simulink library "vmc"  (R2021b)
settings: Solver=VariableStepAuto  StartTime=0.0  StopTime=10.0  RelTol=1e-3
undefined symbols (not defined in the file or in its folder): AVMC_ACCDeltaTqIGain_X_kph, AVMC_ACCDeltaTqIGain_Y_mps2, AVMC_ACCDeltaTqIGainP2_X_kph, AVMC_ACCDeltaTqIGainP2_Y_mps2, AVMC_ACCDeltaTqPGain_X_kph, AVMC_ACCDeltaTqPGain_Y_kph, AVMC_ACCDeltaTqPGainP2_X_kph, AVMC_ACCDeltaTqPGainP2_Y_kph, AVMC_ACCLongSteadyCtrl_X_kph, AVMC_CCAccelCMD_X_kph, AVMC_CCAccelCMD_Y_kph, AVMC_CCDeltaTqIGain_X_kph, AVMC_CCDeltaTqIGain_Y_mps2, AVMC_CCDeltaTqPGain_X_kph, AVMC_CCDeltaTqPGain_Y_kph, AVMC_CCLongSteadyCtrl_X_kph, AVMC_DISCDeltaTqIGainP2_X_kph, AVMC_DISCDeltaTqIGainP2_Y_mps2, AVMC_ESCRegenOut_X_kph, AVMC_ESCRegenOut_Y_Deg, AVMC_ESCRegenOutEnSpd_X_Deg, AVMC_LatESCRegenOut_X_kph, AVMC_LatESCRegenOut_Y_Deg, AVMC_LongAccDeadZone_X_kph, AVMC_LongAccDeadZoneP2_X_kph, AVMC_LongAccFiltTs_X_Gps, AVMC_LongAccFiltTsP2_X_Gps, AVMC_MCPresBaseTq_X_bar, AVMC_MSAAccelCMD_X_kph, AVMC_MSAAccelCMD_Y_kph, AVMC_MSADeltaTqIGain_X_kph, AVMC_MSADeltaTqIGain_Y_mps2, AVMC_MSADeltaTqPGain_X_kph, AVMC_MSADeltaTqPGain_Y_kph, AVMC_MSALongSteadyCtrl_X_kph, AVMC_MSAPedalOvrd_X_kph, AVMC_MSASpdBand_X_kph, AVMC_OPDDisSlideRate_X_Deg, AVMC_RDCDetectTime_X_kph, AVMC_RDCDetectTime_Y_pct, AVMC_RDCEnSlideRate_X_Deg, AVMC_StESCYaw_X_kph, AVMC_StESCYaw_Y_Deg, AVMC_StESCYawCom_X_kph, AVMC_StESCYawCom_Y_Gps, AVMC_TMSpdBaseTq_X_rpm, C_TASK_10MS_S, C_TASK_5MS_S, DEG2RAD, Discrete, ENUM_ADASACCSTA_ACTIVE, ENUM_ADASACCSTA_OVERRIDE, ENUM_ADASACCSTA_STANDBY, ENUM_ADASMSASTA_ACTIVE, ENUM_ADASMSASTA_ERROR, ENUM_ADASMSASTA_OFF, ENUM_ADASMSASTA_OVERSPEED, ENUM_ADASMSASTA_STANDBY, ENUM_ADASMSASTA_UNDERSPEED, ENUM_ADASMSASTA_UNLIMIT ... (+254)
libraries: hcu_lib x57, simulink x49, ctrlSharedLib x6, simulink_extras x1
(part 8 of 9)

== system vmc/VMC/Slide Rate  Calculation/4Wheel Calculation/LR Wheel ==
  VVMC_4WheelLongAcc_Gps : Inport
  task_time_s : Inport  Port=2
  VINP_LRRawWhlSpeed_kph : Inport  Port=3
  VTQD_GearActualPosn_enum : Inport  Port=4
  AND3 : Logic  Inputs=3  AllPortsSameDT=off  OutDataTypeStr=boolean
  Abs2 : Abs
  Add : Sum
  Add{4,7,13..14} (4 alike) : Sum  Inputs=+-
  Constant1 : Constant  Value=GRAVITY_G
  Constant11 : Constant  Value=KPH2MPS
  Constant19 : Constant  Value=ONE_PERCENT
  Constant2 : Constant  Value=MPS2KPH
  Constant20 : Constant  Value=KVMC_RawWhlSpeedDeadZone_kph
  Constant21 : Constant  Value=ZERO_FLOAT
  Constant22 : Constant  Value=KVMC_RawWhlSpeedDeadZone_kph
  Constant23 : Constant  Value=ONE_FLOAT
  Constant30 : Constant  Value=KPH2MPS
  Constant31 : Constant  Value=GRAVITY_G
  Constant32 : Constant  Value=KVMC_WhlSpdCalAccTs_c
  Constant40 : Constant  Value=KVMC_WheelSkidAccDev_Gps
  Constant41 : Constant  Value=KVMC_SkidRecVehSpdDev_kph
  Constant44 : Constant  Value=KPH2MPS
  Constant46 : Constant  Value=ENUM_GEARACTUALPOSN_D
  Constant47 : Constant  Value=ENUM_GEARACTUALPOSN_R
  Constant48 : Constant  Value=KVMC_PreVehSpdCalSW_flg
  Constant5 : Constant  Value=KVMC_4WheelEnSkidDetSpd_kph
  Constant50 : Constant  Value=KVMC_LRWhlSkidReset_flg
  Delay{,3,5,10..11,16} (6 alike) : Delay  DelayLength=1
  Divide4 : Product  Inputs=*//
  Divide6 : Product  Inputs=**//
  Equal : RelationalOperator  Operator===  OutDataTypeStr=boolean  RndMeth=Simplest
  Equal1 : RelationalOperator  Operator===  OutDataTypeStr=boolean  RndMeth=Simplest
  FirstOrderFilter2 : hcu_lib/Basic_Blocks/FirstOrderFilter
  OR : Logic  Operator=OR  AllPortsSameDT=off  OutDataTypeStr=boolean
  OR1 : Logic  Operator=OR  AllPortsSameDT=off  OutDataTypeStr=boolean
  OR2 : Logic  Operator=OR  AllPortsSameDT=off  OutDataTypeStr=boolean
  Product : Product
  Product1 : Product  Inputs=3
  Product2 : Product
  Product3 : Product
  Relational Operator12 : RelationalOperator  Operator=>  OutDataTypeStr=boolean  RndMeth=Simplest
  Relational Operator{2,7..8,13} (4 alike) : RelationalOperator  Operator=<=  OutDataTypeStr=boolean  RndMeth=Simplest
  SR_Latch2 : hcu_lib/Basic_Blocks/SR_Latch
  Saturation : Saturate  UpperLimit=KVMC_PredVehSpdLimit_mps  LowerLimit=ZERO_FLOAT
  Switch{,7..8,10} (4 alike) : Switch  Criteria=u2 > Threshold
  VVMC_LRPreVehSpd_kph : Outport
  VVMC_LRWhlSkid_flg : Outport  Port=2
  VVMC_LR4WhlSpdSlideRate_pct : Outport  Port=3
  wires:
  Delay3/1 -> Add7/2
  Delay10/1 -> Add13/1
  Constant30/1 -> Divide6/2
  [task_time_s] -> Divide6/3
  Constant41/1 -> Relational Operator13/2
  Constant50/1 -> AND3/3
  Constant31/1 -> Divide6/4
  [VINP_LRRawWhlSpeed_kph] -> Delay11/1
  SR_Latch2/1 -> [VVMC_LRWhlSkid_flg]  "VVMC_LRWhlSkid_flg"
  [VVMC_LRWhlSkid_flg] -> Delay16/1
  Relational Operator13/1 -> AND3/1
  Abs2/1 -> Relational Operator13/1
  Delay16/1 -> AND3/2
  Add7/1 -> Divide6/1
  Relational Operator12/1 -> SR_Latch2/1
  Delay11/1 -> Add13/2
  [VINP_LRRawWhlSpeed_kph] -> Add7/1
  [VINP_LRRawWhlSpeed_kph] -> Delay3/1
  [VVMC_LRWhlCalAcc_Gps] -> Add14/1
  Constant32/1 -> FirstOrderFilter2/3
  FirstOrderFilter2/1 -> [VVMC_LRWhlCalAcc_Gps]  "VVMC_LRWhlCalAcc_Gps"
  Divide6/1 -> FirstOrderFilter2/1
  [VVMC_4WheelLongAcc_Gps] -> Add14/2
  Constant40/1 -> Relational Operator12/2
  Add13/1 -> Abs2/1
  Add14/1 -> Relational Operator12/1
  [task_time_s] -> FirstOrderFilter2/2
  [VVMC_LRPreVehSpd_kph] -> Delay5/1
  [task_time_s] -> Product1/3
  [VVMC_4WheelLongAcc_Gps] -> Product1/1
  Constant44/1 -> Product3/2
  Switch/1 -> Saturation/1  "VVMC_LRLastPreVehSpd_mps"
  Product2/1 -> Switch10/1
  Constant11/1 -> Product/2
  Add/1 -> Product2/1  "VVMC_LRCalPreVehSpd_mps"
  Equal/1 -> OR/1
  [VTQD_GearActualPosn_enum] -> Equal/1
  [VINP_LRRawWhlSpeed_kph] -> Switch10/3
  Constant1/1 -> Product1/2
  Product3/1 -> Switch/1
  Switch10/1 -> [VVMC_LRPreVehSpd_kph]  "VVMC_LRPreVehSpd_kph"
  [VINP_LRRawWhlSpeed_kph] -> Delay/1
  OR1/1 -> Switch/2
  Constant48/1 -> OR1/2
  Constant47/1 -> Equal1/2
  Equal1/1 -> OR/2
  [VTQD_GearActualPosn_enum] -> Equal1/1
  Constant46/1 -> Equal/2
  Constant2/1 -> Product2/2
  Product1/1 -> Add/1  "VVMC_LRDeltaVehSpd_mps"
  Delay/1 -> Product/1
  Product/1 -> Switch/3
  Delay5/1 -> Product3/1
  Saturation/1 -> Add/2
  OR/1 -> Switch10/2
  [VVMC_LRWhlSkid_flg] -> OR1/1
  [VVMC_LRPreVehSpd_kph] -> Delay10/1
  Constant22/1 -> Relational Operator7/2
  [VINP_LRRawWhlSpeed_kph] -> Add4/1
  [VINP_LRRawWhlSpeed_kph] -> Relational Operator8/1
  Relational Operator7/1 -> Switch7/2
  [VVMC_LRPreVehSpd_kph] -> Relational Operator7/1
  Constant19/1 -> Divide4/2
  Switch8/1 -> [VVMC_LR4WhlSpdSlideRate_pct]  "VVMC_LR4WhlSpdSlideRate_pct"
  Constant23/1 -> Switch7/1
  [VVMC_LRPreVehSpd_kph] -> Add4/2
  Constant20/1 -> Relational Operator8/2
  Constant21/1 -> Switch8/1
  Divide4/1 -> Switch8/3  "VVMC_LRCal4WhlSpdSlideRate_pct"
  Switch7/1 -> Divide4/3
  [VVMC_LRPreVehSpd_kph] -> Switch7/3
  Add4/1 -> Divide4/1
  Relational Operator8/1 -> Switch8/2
  task_time_s/1 -> [task_time_s]
  VVMC_4WheelLongAcc_Gps/1 -> [VVMC_4WheelLongAcc_Gps]
  VINP_LRRawWhlSpeed_kph/1 -> [VINP_LRRawWhlSpeed_kph]
  VTQD_GearActualPosn_enum/1 -> [VTQD_GearActualPosn_enum]
  [VVMC_LRPreVehSpd_kph] -> VVMC_LRPreVehSpd_kph/1
  [VVMC_LRWhlSkid_flg] -> VVMC_LRWhlSkid_flg/1
  [VVMC_LR4WhlSpdSlideRate_pct] -> VVMC_LR4WhlSpdSlideRate_pct/1
  [VINP_LRRawWhlSpeed_kph] -> Relational Operator2/1
  Relational Operator2/1 -> OR2/1
  Constant5/1 -> Relational Operator2/2
  AND3/1 -> OR2/2
  OR2/1 -> SR_Latch2/2  "VVMC_LRWhlSkidReset_flg"

== system vmc/VMC/Slide Rate  Calculation/4Wheel Calculation/RF Wheel ==
  VVMC_4WheelLongAcc_Gps : Inport
  task_time_s : Inport  Port=2
  VINP_RFRawWhlSpeed_kph : Inport  Port=3
  VTQD_GearActualPosn_enum : Inport  Port=4
  AND2 : Logic  Inputs=3  AllPortsSameDT=off  OutDataTypeStr=boolean
  Abs1 : Abs
  Add : Sum
  Add{2,6,11..12} (4 alike) : Sum  Inputs=+-
  Constant1 : Constant  Value=GRAVITY_G
  Constant10 : Constant  Value=ONE_PERCENT
  Constant11 : Constant  Value=KPH2MPS
  Constant12 : Constant  Value=KVMC_RawWhlSpeedDeadZone_kph
  Constant13 : Constant  Value=ZERO_FLOAT
  Constant2 : Constant  Value=MPS2KPH
  Constant27 : Constant  Value=KPH2MPS
  Constant28 : Constant  Value=GRAVITY_G
  Constant29 : Constant  Value=KVMC_WhlSpdCalAccTs_c
  Constant3 : Constant  Value=KVMC_RawWhlSpeedDeadZone_kph
  Constant38 : Constant  Value=KVMC_WheelSkidAccDev_Gps
  Constant39 : Constant  Value=KVMC_SkidRecVehSpdDev_kph
  Constant4 : Constant  Value=ONE_FLOAT
  Constant44 : Constant  Value=KPH2MPS
  Constant46 : Constant  Value=ENUM_GEARACTUALPOSN_D
  Constant47 : Constant  Value=ENUM_GEARACTUALPOSN_R
  Constant48 : Constant  Value=KVMC_PreVehSpdCalSW_flg
  Constant5 : Constant  Value=KVMC_4WheelEnSkidDetSpd_kph
  Constant51 : Constant  Value=KVMC_RFWhlSkidReset_flg
  Delay{,2,5,8..9,15} (6 alike) : Delay  DelayLength=1
  Divide2 : Product  Inputs=*//
  Divide5 : Product  Inputs=**//
  Equal : RelationalOperator  Operator===  OutDataTypeStr=boolean  RndMeth=Simplest
  Equal1 : RelationalOperator  Operator===  OutDataTypeStr=boolean  RndMeth=Simplest
  FirstOrderFilter1 : hcu_lib/Basic_Blocks/FirstOrderFilter
  OR : Logic  Operator=OR  AllPortsSameDT=off  OutDataTypeStr=boolean
  OR1 : Logic  Operator=OR  AllPortsSameDT=off  OutDataTypeStr=boolean
  OR2 : Logic  Operator=OR  AllPortsSameDT=off  OutDataTypeStr=boolean
  Product : Product
  Product1 : Product  Inputs=3
  Product2 : Product
  Product3 : Product
  Relational Operator{1..2,4,11} (4 alike) : RelationalOperator  Operator=<=  OutDataTypeStr=boolean  RndMeth=Simplest
  Relational Operator10 : RelationalOperator  Operator=>  OutDataTypeStr=boolean  RndMeth=Simplest
  SR_Latch1 : hcu_lib/Basic_Blocks/SR_Latch
  Saturation : Saturate  UpperLimit=KVMC_PredVehSpdLimit_mps  LowerLimit=ZERO_FLOAT
  Switch{,1,4,10} (4 alike) : Switch  Criteria=u2 > Threshold
  VVMC_RFPreVehSpd_kph : Outport
  VVMC_RFWhlSkid_flg : Outport  Port=2
  VVMC_RF4WhlSpdSlideRate_pct : Outport  Port=3
  wires:
  [VVMC_4WheelLongAcc_Gps] -> Add12/2
  Switch1/1 -> Divide2/3
  Relational Operator11/1 -> AND2/1
  Divide5/1 -> FirstOrderFilter1/1
  Constant12/1 -> Relational Operator4/2
  Add12/1 -> Relational Operator10/1
  [VINP_RFRawWhlSpeed_kph] -> Add6/1
  Constant13/1 -> Switch4/1
  [VINP_RFRawWhlSpeed_kph] -> Delay2/1
  Constant3/1 -> Relational Operator1/2
  Delay15/1 -> AND2/2
  [VVMC_RFWhlSkid_flg] -> Delay15/1
  Constant27/1 -> Divide5/2
  Relational Operator1/1 -> Switch1/2
  Constant28/1 -> Divide5/4
  Add11/1 -> Abs1/1
  Constant38/1 -> Relational Operator10/2
  Divide2/1 -> Switch4/3  "VVMC_RFCal4WhlSpdSlideRate_pct"
  Delay8/1 -> Add11/1
  [VINP_RFRawWhlSpeed_kph] -> Delay9/1
  Abs1/1 -> Relational Operator11/1
  [task_time_s] -> FirstOrderFilter1/2
  Delay9/1 -> Add11/2
  Constant39/1 -> Relational Operator11/2
  Constant4/1 -> Switch1/1
  Relational Operator4/1 -> Switch4/2
  Constant51/1 -> AND2/3
  Add6/1 -> Divide5/1
  Constant10/1 -> Divide2/2
  [VINP_RFRawWhlSpeed_kph] -> Add2/1
  [VINP_RFRawWhlSpeed_kph] -> Relational Operator4/1
  Relational Operator10/1 -> SR_Latch1/1
  SR_Latch1/1 -> [VVMC_RFWhlSkid_flg]  "VVMC_RFWhlSkid_flg"
  [VVMC_RFWhlCalAcc_Gps] -> Add12/1
  Constant29/1 -> FirstOrderFilter1/3
  FirstOrderFilter1/1 -> [VVMC_RFWhlCalAcc_Gps]  "VVMC_RFWhlCalAcc_Gps"
  Switch4/1 -> [VVMC_RF4WhlSpdSlideRate_pct]  "VVMC_RF4WhlSpdSlideRate_pct"
  Add2/1 -> Divide2/1
  Delay2/1 -> Add6/2
  [task_time_s] -> Divide5/3
  Product/1 -> Switch/3
  Delay5/1 -> Product3/1
  Product3/1 -> Switch/1
  [VVMC_RFPreVehSpd_kph] -> Delay5/1
  [VINP_RFRawWhlSpeed_kph] -> Delay/1
  OR/1 -> Switch10/2
  [VTQD_GearActualPosn_enum] -> Equal/1
  [VINP_RFRawWhlSpeed_kph] -> Switch10/3
  [VTQD_GearActualPosn_enum] -> Equal1/1
  Delay/1 -> Product/1
  Saturation/1 -> Add/2
  Constant2/1 -> Product2/2
  Product1/1 -> Add/1  "VVMC_RFDeltaVehSpd_mps"
  Equal1/1 -> OR/2
  Constant46/1 -> Equal/2
  OR1/1 -> Switch/2
  Constant47/1 -> Equal1/2
  Constant48/1 -> OR1/2
  Switch10/1 -> [VVMC_RFPreVehSpd_kph]  "VVMC_RFPreVehSpd_kph"
  Constant1/1 -> Product1/2
  Product2/1 -> Switch10/1
  Constant11/1 -> Product/2
  Switch/1 -> Saturation/1  "VVMC_RFLastPreVehSpd_mps"
  Constant44/1 -> Product3/2
  [VVMC_4WheelLongAcc_Gps] -> Product1/1
  [task_time_s] -> Product1/3
  Equal/1 -> OR/1
  Add/1 -> Product2/1  "VVMC_RFCalPreVehSpd_mps"
  [VVMC_RFWhlSkid_flg] -> OR1/1
  [VVMC_RFPreVehSpd_kph] -> Delay8/1
  [VVMC_RFPreVehSpd_kph] -> Add2/2
  [VVMC_RFPreVehSpd_kph] -> Relational Operator1/1
  [VVMC_RFPreVehSpd_kph] -> Switch1/3
  VTQD_GearActualPosn_enum/1 -> [VTQD_GearActualPosn_enum]
  VINP_RFRawWhlSpeed_kph/1 -> [VINP_RFRawWhlSpeed_kph]
  VVMC_4WheelLongAcc_Gps/1 -> [VVMC_4WheelLongAcc_Gps]
  task_time_s/1 -> [task_time_s]
  [VVMC_RFPreVehSpd_kph] -> VVMC_RFPreVehSpd_kph/1
  [VVMC_RFWhlSkid_flg] -> VVMC_RFWhlSkid_flg/1
  [VVMC_RF4WhlSpdSlideRate_pct] -> VVMC_RF4WhlSpdSlideRate_pct/1
  Constant5/1 -> Relational Operator2/2
  Relational Operator2/1 -> OR2/1
  [VINP_RFRawWhlSpeed_kph] -> Relational Operator2/1
  AND2/1 -> OR2/2
  OR2/1 -> SR_Latch1/2  "VVMC_RFWhlSkidReset_flg"

== system vmc/VMC/Slide Rate  Calculation/4Wheel Calculation/RR Wheel ==
  VVMC_4WheelLongAcc_Gps : Inport
  task_time_s : Inport  Port=2
  VINP_RRRawWhlSpeed_kph : Inport  Port=3
  VTQD_GearActualPosn_enum : Inport  Port=4
  AND4 : Logic  Inputs=3  AllPortsSameDT=off  OutDataTypeStr=boolean
  Abs3 : Abs
  Add : Sum
  Add{3,8,15..16} (4 alike) : Sum  Inputs=+-
  Constant1 : Constant  Value=GRAVITY_G
  Constant11 : Constant  Value=KPH2MPS
  Constant14 : Constant  Value=ONE_PERCENT
  Constant15 : Constant  Value=KVMC_RawWhlSpeedDeadZone_kph
  Constant16 : Constant  Value=ZERO_FLOAT
  Constant17 : Constant  Value=KVMC_RawWhlSpeedDeadZone_kph
  Constant18 : Constant  Value=ONE_FLOAT
  Constant2 : Constant  Value=MPS2KPH
  Constant33 : Constant  Value=KPH2MPS
  Constant34 : Constant  Value=GRAVITY_G
  Constant35 : Constant  Value=KVMC_WhlSpdCalAccTs_c
  Constant42 : Constant  Value=KVMC_WheelSkidAccDev_Gps
  Constant43 : Constant  Value=KVMC_SkidRecVehSpdDev_kph
  Constant44 : Constant  Value=KPH2MPS
  Constant46 : Constant  Value=ENUM_GEARACTUALPOSN_D
  Constant47 : Constant  Value=ENUM_GEARACTUALPOSN_R
  Constant48 : Constant  Value=KVMC_PreVehSpdCalSW_flg
  Constant49 : Constant  Value=KVMC_RRWhlSkidReset_flg
  Constant5 : Constant  Value=KVMC_4WheelEnSkidDetSpd_kph
  Delay{,4..5,12..13,17} (6 alike) : Delay  DelayLength=1
  Divide3 : Product  Inputs=*//
  Divide7 : Product  Inputs=**//
  Equal : RelationalOperator  Operator===  OutDataTypeStr=boolean  RndMeth=Simplest
  Equal1 : RelationalOperator  Operator===  OutDataTypeStr=boolean  RndMeth=Simplest
  FirstOrderFilter3 : hcu_lib/Basic_Blocks/FirstOrderFilter
  OR : Logic  Operator=OR  AllPortsSameDT=off  OutDataTypeStr=boolean
  OR1 : Logic  Operator=OR  AllPortsSameDT=off  OutDataTypeStr=boolean
  OR2 : Logic  Operator=OR  AllPortsSameDT=off  OutDataTypeStr=boolean
  Product : Product
  Product1 : Product  Inputs=3
  Product2 : Product
  Product3 : Product
  Relational Operator14 : RelationalOperator  Operator=>  OutDataTypeStr=boolean  RndMeth=Simplest
  Relational Operator{2,5..6,15} (4 alike) : RelationalOperator  Operator=<=  OutDataTypeStr=boolean  RndMeth=Simplest
  SR_Latch3 : hcu_lib/Basic_Blocks/SR_Latch
  Saturation : Saturate  UpperLimit=KVMC_PredVehSpdLimit_mps  LowerLimit=ZERO_FLOAT
  Switch{,5..6,10} (4 alike) : Switch  Criteria=u2 > Threshold
  VVMC_RRPreVehSpd_kph : Outport
  VVMC_RRWhlSkid_flg : Outport  Port=2
  VVMC_RR4WhlSpdSlideRate_pct : Outport  Port=3
  wires:
  [VINP_RRRawWhlSpeed_kph] -> Add8/1
  Constant49/1 -> AND4/3
  Add8/1 -> Divide7/1
  [task_time_s] -> Divide7/3
  Add15/1 -> Abs3/1
  Relational Operator14/1 -> SR_Latch3/1
  [VVMC_4WheelLongAcc_Gps] -> Add16/2
  [task_time_s] -> FirstOrderFilter3/2
  [VINP_RRRawWhlSpeed_kph] -> Delay4/1
  Constant42/1 -> Relational Operator14/2
  FirstOrderFilter3/1 -> [VVMC_RRWhlCalAcc_Gps]  "VVMC_RRWhlCalAcc_Gps"
  Divide7/1 -> FirstOrderFilter3/1
  Relational Operator15/1 -> AND4/1
  Delay4/1 -> Add8/2
  Delay17/1 -> AND4/2
  [VVMC_RRWhlSkid_flg] -> Delay17/1
  Add16/1 -> Relational Operator14/1
  Delay12/1 -> Add15/1
  Constant43/1 -> Relational Operator15/2
  Delay13/1 -> Add15/2
  Constant33/1 -> Divide7/2
  Constant34/1 -> Divide7/4
  Abs3/1 -> Relational Operator15/1
  SR_Latch3/1 -> [VVMC_RRWhlSkid_flg]  "VVMC_RRWhlSkid_flg"
  [VVMC_RRWhlCalAcc_Gps] -> Add16/1
  Constant35/1 -> FirstOrderFilter3/3
  Constant14/1 -> Divide3/2
  Switch5/1 -> Divide3/3
  Divide3/1 -> Switch6/3  "VVMC_RRCal4WhlSpdSlideRate_pct"
  Switch6/1 -> [VVMC_RR4WhlSpdSlideRate_pct]  "VVMC_RR4WhlSpdSlideRate_pct"
  Constant18/1 -> Switch5/1
  Relational Operator6/1 -> Switch6/2
  [VINP_RRRawWhlSpeed_kph] -> Relational Operator6/1
  Relational Operator5/1 -> Switch5/2
  Constant15/1 -> Relational Operator6/2
  Constant16/1 -> Switch6/1
  Constant17/1 -> Relational Operator5/2
  [VINP_RRRawWhlSpeed_kph] -> Add3/1
  Add3/1 -> Divide3/1
  Product3/1 -> Switch/1
  Constant1/1 -> Product1/2
  Switch10/1 -> [VVMC_RRPreVehSpd_kph]  "VVMC_RRPreVehSpd_kph"
  [VINP_RRRawWhlSpeed_kph] -> Switch10/3
  [VTQD_GearActualPosn_enum] -> Equal/1
  Add/1 -> Product2/1  "VVMC_RRCalPreVehSpd_mps"
  Equal/1 -> OR/1
  Product2/1 -> Switch10/1
  [VVMC_4WheelLongAcc_Gps] -> Product1/1
  Constant11/1 -> Product/2
  Constant44/1 -> Product3/2
  [task_time_s] -> Product1/3
  Switch/1 -> Saturation/1  "VVMC_RRLastPreVehSpd_mps"
  [VVMC_RRPreVehSpd_kph] -> Delay5/1
  Delay/1 -> Product/1
  Constant47/1 -> Equal1/2
  Equal1/1 -> OR/2
  [VTQD_GearActualPosn_enum] -> Equal1/1
  Constant48/1 -> OR1/2
  Constant2/1 -> Product2/2
  OR1/1 -> Switch/2
  Constant46/1 -> Equal/2
  Product1/1 -> Add/1  "VVMC_RRDeltaVehSpd_mps"
  Saturation/1 -> Add/2
  Delay5/1 -> Product3/1
  Product/1 -> Switch/3
  OR/1 -> Switch10/2
  [VVMC_RRWhlSkid_flg] -> OR1/1
  [VINP_RRRawWhlSpeed_kph] -> Delay/1
  [VINP_RRRawWhlSpeed_kph] -> Delay13/1
  [VVMC_RRPreVehSpd_kph] -> Delay12/1
  [VVMC_RRPreVehSpd_kph] -> Add3/2
  [VVMC_RRPreVehSpd_kph] -> Relational Operator5/1
  [VVMC_RRPreVehSpd_kph] -> Switch5/3
  VVMC_4WheelLongAcc_Gps/1 -> [VVMC_4WheelLongAcc_Gps]
  VTQD_GearActualPosn_enum/1 -> [VTQD_GearActualPosn_enum]
  task_time_s/1 -> [task_time_s]
  VINP_RRRawWhlSpeed_kph/1 -> [VINP_RRRawWhlSpeed_kph]
  [VVMC_RRPreVehSpd_kph] -> VVMC_RRPreVehSpd_kph/1
  [VVMC_RRWhlSkid_flg] -> VVMC_RRWhlSkid_flg/1
  [VVMC_RR4WhlSpdSlideRate_pct] -> VVMC_RR4WhlSpdSlideRate_pct/1
  Constant5/1 -> Relational Operator2/2
  [VINP_RRRawWhlSpeed_kph] -> Relational Operator2/1
  Relational Operator2/1 -> OR2/1
  AND4/1 -> OR2/2
  OR2/1 -> SR_Latch3/2  "VVMC_RRWhlSkidReset_flg"

== system vmc/VMC/ACC_Function/ACC Delta Torque Map and Calculation/Phase2_ADASWhlTqCal/Triggered Subsystem1 ==
  In1 : Inport
  In2 : Inport  Port=2
  In3 : Inport  Port=3
  Trigger : TriggerPort  VariantControl=(inherit)
  Out1 : Outport
  Out2 : Outport  Port=2
  Out3 : Outport  Port=3
  wires:
  In1/1 -> Out1/1
  In2/1 -> Out2/1
  In3/1 -> Out3/1

== system vmc/VMC/ACC_Function/ACC Delta Torque Map and Calculation/Phase2_ADASWhlTqCal/Triggered Subsystem2 ==
  In1 : Inport
  Trigger : TriggerPort  VariantControl=(inherit)
  Out1 : Outport
  wires:
  In1/1 -> Out1/1

== system vmc/VMC/ACC_Function/ACC Delta Torque Map and Calculation/Phase2_ADASWhlTqCal/Triggered Subsystem4 ==
  In1 : Inport
  In2 : Inport  Port=2
  Trigger : TriggerPort  VariantControl=(inherit)
  Out1 : Outport
  Out2 : Outport  Port=2
  wires:
  In1/1 -> Out1/1
  In2/1 -> Out2/1

== system vmc/VMC/ACC_Function/ACC Delta Torque Map and Calculation/Phase2_ADASWhlTqCal/Triggered Subsystem5 ==
  In1 : Inport
  Trigger : TriggerPort  VariantControl=(inherit)
  Out1 : Outport
  wires:
  In1/1 -> Out1/1

== stateflow chart vmc/VMC/IMU/IMU sensing result /RollingAverage3 ==
  state RollingAverage
    (default) -> (junction 2) : {VVMC_RollAveCount_enum = ONE_INT}
    RollingAverage -> (junction 2)
    (junction 2) -> (junction 3) : {VVMC_RollAve_raw32 = ZERO_FLOAT}
    (junction 3) -> (junction 100) [order 1] : [VVMC_RollAveCount_enum < KVMC_RollAveLevel_enum]
    (junction 3) -> (junction 37) [order 2]
    (junction 100) -> (junction 5) : {% Memory
        |  VVMC_Memory_raw32[VVMC_RollAveCount_enum] = VINP_INPData_raw32;
        |
        |  % Memory Shift Counter
        |  VVMC_ShiftCount_enum = ONE_INT}
    (junction 5) -> (junction 7) [order 2]
    (junction 5) -> (junction 6) [order 1] : [VVMC_ShiftCount_enum <= VVMC_RollAveCount_enum]
    (junction 7) -> (junction 8) : {% Rolling Average
        |  VVMC_RollAve_raw32 = VVMC_RollAve_raw32 / VVMC_RollAveCount_enum;
        |
        |  % Rolling Average Counter
        |  VVMC_RollAveCount_enum++}
    (junction 35) -> (junction 5) : {VVMC_ShiftCount_enum++}
    (junction 6) -> (junction 36) : {% Rolling Average Sum
        |  VVMC_RollAve_raw32 = VVMC_RollAve_raw32 + VVMC_Memory_raw32[VVMC_ShiftCount_enum];
        |  }
    (junction 36) -> (junction 35)
    (junction 37) -> (junction 76) [order 1] : [VVMC_RollAveCount_enum == KVMC_RollAveLevel_enum]
    (junction 76) -> (junction 47)
    (junction 37) -> (junction 60) [order 2]
    (junction 78) -> (junction 76)
    (junction 47) -> (junction 30) : {% Memory
        |  VVMC_Memory_raw32[VVMC_RollAveCount_enum] = VINP_INPData_raw32;
        |
        |  % Memory Shift Counter
        |  VVMC_ShiftCount_enum = ONE_INT;
        | }
    (junction 60) -> (junction 62) [order 1] : [VVMC_RollAveCount_enum > KVMC_RollAveLevel_enum]
    (junction 60) -> (junction 39) [order 2]
    (junction 62) -> (junction 66) : {VVMC_MemoryShiftCount_enum = ONE_INT}
    (junction 30) -> (junction 48) [order 2]
    (junction 30) -> (junction 22) [order 1] : [VVMC_ShiftCount_enum <= VVMC_RollAveCount_enum]
    (junction 48) -> (junction 45) : {% Rolling Average
        |  VVMC_RollAve_raw32 = VVMC_RollAve_raw32 / VVMC_RollAveCount_enum;
        |
        |  % Memory Shift Counter
        |  VVMC_ShiftCount_enum = ONE_INT}
    (junction 14) -> (junction 30) : {VVMC_ShiftCount_enum++}
    (junction 22) -> (junction 25) : {% Rolling Average Sum
        |  VVMC_RollAve_raw32 = VVMC_RollAve_raw32 + VVMC_Memory_raw32[VVMC_ShiftCount_enum]}
    (junction 66) -> (junction 82) [order 2]
    (junction 66) -> (junction 69) [order 1] : [VVMC_MemoryShiftCount_enum < VVMC_RollAveCount_enum]
    (junction 82) -> (junction 80) : {VVMC_RollAveCount_enum = KVMC_RollAveLevel_enum}
    (junction 73) -> (junction 66) : {VVMC_MemoryShiftCount_enum++}
    (junction 69) -> (junction 71) : {VVMC_Memory_raw32[VVMC_MemoryShiftCount_enum] =...
        |  VVMC_Memory_raw32[VVMC_RollAveCount_enum - KVMC_RollAveLevel_enum + VVMC_MemoryShiftCount_enum]}
    (junction 25) -> (junction 14)
    (junction 71) -> (junction 73)
    (junction 80) -> (junction 78)
    (junction 45) -> (junction 39) [order 2]
    (junction 45) -> (junction 15) [order 1] : [VVMC_ShiftCount_enum < VVMC_RollAveCount_enum]
    (junction 41) -> (junction 45) : { VVMC_ShiftCount_enum++}
    (junction 15) -> (junction 38) : {% Gy Memory Shift
        |  VVMC_Memory_raw32[VVMC_ShiftCount_enum] = VVMC_Memory_raw32[VVMC_ShiftCount_enum + ONE_INT]}
    (junction 38) -> (junction 41)
  data: KVMC_RollAveLevel_enum input uint8; VVMC_ShiftCount_enum local uint8; VVMC_RollAveCount_enum local uint8; VVMC_Memory_raw32 local single size=256; ZERO_FLOAT input single; ONE_INT input uint8; VVMC_RollAve_raw32 output single; VINP_INPData_raw32 input single; VVMC_MemoryShiftCount_enum local uint8

== stateflow chart vmc/VMC/LongAccel_EstSlope/VehSpdRollingAverage/RollingAverage ==
  state LatAccelRollingAverage
    (default) -> (junction 2) : {VVMC_RollAveCount_enum = ONE_INT}
    LatAccelRollingAverage -> (junction 2)
    (junction 2) -> (junction 3) : {VVMC_VehSpdRollAve_kph = ZERO_FLOAT}
    (junction 3) -> (junction 100) [order 1] : [VVMC_RollAveCount_enum < KVMC_VehSpdRollAveLevel_enum]
    (junction 3) -> (junction 37) [order 2]
    (junction 100) -> (junction 5) : {% Memory
        |  VVMC_Memory_raw32[VVMC_RollAveCount_enum] = VINP_VehSpeed_kph;
        |
        |  % Memory Shift Counter
        |  VVMC_ShiftCount_enum = ONE_INT}
    (junction 5) -> (junction 7) [order 2]
    (junction 5) -> (junction 6) [order 1] : [VVMC_ShiftCount_enum <= VVMC_RollAveCount_enum]
    (junction 7) -> (junction 8) : {% Rolling Average
        |  VVMC_VehSpdRollAve_kph = VVMC_VehSpdRollAve_kph / VVMC_RollAveCount_enum;
        |
        |  % Rolling Average Counter
        |  VVMC_RollAveCount_enum++}
    (junction 35) -> (junction 5) : {VVMC_ShiftCount_enum++}
    (junction 6) -> (junction 36) : {% Rolling Average Sum
        |  VVMC_VehSpdRollAve_kph = VVMC_VehSpdRollAve_kph + VVMC_Memory_raw32[VVMC_ShiftCount_enum];
        |  }
    (junction 36) -> (junction 35)
    (junction 37) -> (junction 76) [order 1] : [VVMC_RollAveCount_enum == KVMC_VehSpdRollAveLevel_enum]
    (junction 76) -> (junction 47)
    (junction 37) -> (junction 60) [order 2]
    (junction 78) -> (junction 76)
    (junction 47) -> (junction 30) : {% Memory
        |  VVMC_Memory_raw32[VVMC_RollAveCount_enum] = VINP_VehSpeed_kph;
        |
        |  % Memory Shift Counter
        |  VVMC_ShiftCount_enum = ONE_INT;
        | }
    (junction 60) -> (junction 62) [order 1] : [VVMC_RollAveCount_enum > KVMC_VehSpdRollAveLevel_enum]
    (junction 60) -> (junction 39) [order 2]
    (junction 62) -> (junction 66) : {VVMC_MemoryShiftCount_enum = ONE_INT}
    (junction 30) -> (junction 48) [order 2]
    (junction 30) -> (junction 22) [order 1] : [VVMC_ShiftCount_enum <= VVMC_RollAveCount_enum]
    (junction 48) -> (junction 45) : {% Rolling Average
        |  VVMC_VehSpdRollAve_kph = VVMC_VehSpdRollAve_kph / VVMC_RollAveCount_enum;
        |
        |  % Memory Shift Counter
        |  VVMC_ShiftCount_enum = ONE_INT}
    (junction 14) -> (junction 30) : {VVMC_ShiftCount_enum++}
    (junction 22) -> (junction 25) : {% Rolling Average Sum
        |  VVMC_VehSpdRollAve_kph = VVMC_VehSpdRollAve_kph + VVMC_Memory_raw32[VVMC_ShiftCount_enum]}
    (junction 66) -> (junction 82) [order 2]
    (junction 66) -> (junction 69) [order 1] : [VVMC_MemoryShiftCount_enum < VVMC_RollAveCount_enum]
    (junction 82) -> (junction 80) : {VVMC_RollAveCount_enum = KVMC_VehSpdRollAveLevel_enum}
    (junction 73) -> (junction 66) : {VVMC_MemoryShiftCount_enum++}
    (junction 69) -> (junction 71) : {VVMC_Memory_raw32[VVMC_MemoryShiftCount_enum] =...
        |  VVMC_Memory_raw32[VVMC_RollAveCount_enum - KVMC_VehSpdRollAveLevel_enum + VVMC_MemoryShiftCount_enum]}
    (junction 25) -> (junction 14)
    (junction 71) -> (junction 73)
    (junction 80) -> (junction 78)
    (junction 45) -> (junction 39) [order 2]
    (junction 45) -> (junction 15) [order 1] : [VVMC_ShiftCount_enum < VVMC_RollAveCount_enum]
    (junction 41) -> (junction 45) : { VVMC_ShiftCount_enum++}
    (junction 15) -> (junction 38) : {% Gy Memory Shift
        |  VVMC_Memory_raw32[VVMC_ShiftCount_enum] = VVMC_Memory_raw32[VVMC_ShiftCount_enum + ONE_INT]}
    (junction 38) -> (junction 41)
  data: KVMC_VehSpdRollAveLevel_enum input uint8; VVMC_ShiftCount_enum local uint8; VVMC_RollAveCount_enum local uint8; VVMC_Memory_raw32 local single size=256; ZERO_FLOAT input single; ONE_INT input uint8; VVMC_VehSpdRollAve_kph output single; VINP_VehSpeed_kph input single; VVMC_MemoryShiftCount_enum local uint8

== stateflow chart vmc/VMC/IMU/IMU sensing result /RollingAverage4 ==
  state RollingAverage
    (default) -> (junction 2) : {VVMC_RollAveCount_enum = ONE_INT}
    RollingAverage -> (junction 2)
    (junction 2) -> (junction 3) : {VVMC_RollAve_raw32 = ZERO_FLOAT}
    (junction 3) -> (junction 100) [order 1] : [VVMC_RollAveCount_enum < KVMC_RollAveLevel_enum]
    (junction 3) -> (junction 37) [order 2]
    (junction 100) -> (junction 5) : {% Memory
        |  VVMC_Memory_raw32[VVMC_RollAveCount_enum] = VINP_INPData_raw32;
        |
        |  % Memory Shift Counter
        |  VVMC_ShiftCount_enum = ONE_INT}
    (junction 5) -> (junction 7) [order 2]
    (junction 5) -> (junction 6) [order 1] : [VVMC_ShiftCount_enum <= VVMC_RollAveCount_enum]
    (junction 7) -> (junction 8) : {% Rolling Average
        |  VVMC_RollAve_raw32 = VVMC_RollAve_raw32 / VVMC_RollAveCount_enum;
        |
        |  % Rolling Average Counter
        |  VVMC_RollAveCount_enum++}
    (junction 35) -> (junction 5) : {VVMC_ShiftCount_enum++}
    (junction 6) -> (junction 36) : {% Rolling Average Sum
        |  VVMC_RollAve_raw32 = VVMC_RollAve_raw32 + VVMC_Memory_raw32[VVMC_ShiftCount_enum];
        |  }
    (junction 36) -> (junction 35)
    (junction 37) -> (junction 76) [order 1] : [VVMC_RollAveCount_enum == KVMC_RollAveLevel_enum]
    (junction 76) -> (junction 47)
    (junction 37) -> (junction 60) [order 2]
    (junction 78) -> (junction 76)
    (junction 47) -> (junction 30) : {% Memory
        |  VVMC_Memory_raw32[VVMC_RollAveCount_enum] = VINP_INPData_raw32;
        |
        |  % Memory Shift Counter
        |  VVMC_ShiftCount_enum = ONE_INT;
        | }
    (junction 60) -> (junction 62) [order 1] : [VVMC_RollAveCount_enum > KVMC_RollAveLevel_enum]
    (junction 60) -> (junction 39) [order 2]
    (junction 62) -> (junction 66) : {VVMC_MemoryShiftCount_enum = ONE_INT}
    (junction 30) -> (junction 48) [order 2]
    (junction 30) -> (junction 22) [order 1] : [VVMC_ShiftCount_enum <= VVMC_RollAveCount_enum]
    (junction 48) -> (junction 45) : {% Rolling Average
        |  VVMC_RollAve_raw32 = VVMC_RollAve_raw32 / VVMC_RollAveCount_enum;
        |
        |  % Memory Shift Counter
        |  VVMC_ShiftCount_enum = ONE_INT}
    (junction 14) -> (junction 30) : {VVMC_ShiftCount_enum++}
    (junction 22) -> (junction 25) : {% Rolling Average Sum
        |  VVMC_RollAve_raw32 = VVMC_RollAve_raw32 + VVMC_Memory_raw32[VVMC_ShiftCount_enum]}
    (junction 66) -> (junction 82) [order 2]
    (junction 66) -> (junction 69) [order 1] : [VVMC_MemoryShiftCount_enum < VVMC_RollAveCount_enum]
    (junction 82) -> (junction 80) : {VVMC_RollAveCount_enum = KVMC_RollAveLevel_enum}
    (junction 73) -> (junction 66) : {VVMC_MemoryShiftCount_enum++}
    (junction 69) -> (junction 71) : {VVMC_Memory_raw32[VVMC_MemoryShiftCount_enum] =...
        |  VVMC_Memory_raw32[VVMC_RollAveCount_enum - KVMC_RollAveLevel_enum + VVMC_MemoryShiftCount_enum]}
    (junction 25) -> (junction 14)
    (junction 71) -> (junction 73)
    (junction 80) -> (junction 78)
    (junction 45) -> (junction 39) [order 2]
    (junction 45) -> (junction 15) [order 1] : [VVMC_ShiftCount_enum < VVMC_RollAveCount_enum]
    (junction 41) -> (junction 45) : { VVMC_ShiftCount_enum++}
    (junction 15) -> (junction 38) : {% Gy Memory Shift
        |  VVMC_Memory_raw32[VVMC_ShiftCount_enum] = VVMC_Memory_raw32[VVMC_ShiftCount_enum + ONE_INT]}
    (junction 38) -> (junction 41)
  data: KVMC_RollAveLevel_enum input uint8; VVMC_ShiftCount_enum local uint8; VVMC_RollAveCount_enum local uint8; VVMC_Memory_raw32 local single size=256; ZERO_FLOAT input single; ONE_INT input uint8; VVMC_RollAve_raw32 output single; VINP_INPData_raw32 input single; VVMC_MemoryShiftCount_enum local uint8

== stateflow chart vmc/VMC/IMU/IMU sensing result /RollingAverage5 ==
  state RollingAverage
    (default) -> (junction 2) : {VVMC_RollAveCount_enum = ONE_INT}
    RollingAverage -> (junction 2)
    (junction 2) -> (junction 3) : {VVMC_RollAve_raw32 = ZERO_FLOAT}
    (junction 3) -> (junction 100) [order 1] : [VVMC_RollAveCount_enum < KVMC_RollAveLevel_enum]
    (junction 3) -> (junction 37) [order 2]
    (junction 100) -> (junction 5) : {% Memory
        |  VVMC_Memory_raw32[VVMC_RollAveCount_enum] = VINP_INPData_raw32;
        |
        |  % Memory Shift Counter
        |  VVMC_ShiftCount_enum = ONE_INT}
    (junction 5) -> (junction 7) [order 2]
    (junction 5) -> (junction 6) [order 1] : [VVMC_ShiftCount_enum <= VVMC_RollAveCount_enum]
    (junction 7) -> (junction 8) : {% Rolling Average
        |  VVMC_RollAve_raw32 = VVMC_RollAve_raw32 / VVMC_RollAveCount_enum;
        |
        |  % Rolling Average Counter
        |  VVMC_RollAveCount_enum++}
    (junction 35) -> (junction 5) : {VVMC_ShiftCount_enum++}
    (junction 6) -> (junction 36) : {% Rolling Average Sum
        |  VVMC_RollAve_raw32 = VVMC_RollAve_raw32 + VVMC_Memory_raw32[VVMC_ShiftCount_enum];
        |  }
    (junction 36) -> (junction 35)
    (junction 37) -> (junction 76) [order 1] : [VVMC_RollAveCount_enum == KVMC_RollAveLevel_enum]
    (junction 76) -> (junction 47)
    (junction 37) -> (junction 60) [order 2]
    (junction 78) -> (junction 76)
    (junction 47) -> (junction 30) : {% Memory
        |  VVMC_Memory_raw32[VVMC_RollAveCount_enum] = VINP_INPData_raw32;
        |
        |  % Memory Shift Counter
        |  VVMC_ShiftCount_enum = ONE_INT;
        | }
    (junction 60) -> (junction 62) [order 1] : [VVMC_RollAveCount_enum > KVMC_RollAveLevel_enum]
    (junction 60) -> (junction 39) [order 2]
    (junction 62) -> (junction 66) : {VVMC_MemoryShiftCount_enum = ONE_INT}
    (junction 30) -> (junction 48) [order 2]
    (junction 30) -> (junction 22) [order 1] : [VVMC_ShiftCount_enum <= VVMC_RollAveCount_enum]
    (junction 48) -> (junction 45) : {% Rolling Average
        |  VVMC_RollAve_raw32 = VVMC_RollAve_raw32 / VVMC_RollAveCount_enum;
        |
        |  % Memory Shift Counter
        |  VVMC_ShiftCount_enum = ONE_INT}
    (junction 14) -> (junction 30) : {VVMC_ShiftCount_enum++}
    (junction 22) -> (junction 25) : {% Rolling Average Sum
        |  VVMC_RollAve_raw32 = VVMC_RollAve_raw32 + VVMC_Memory_raw32[VVMC_ShiftCount_enum]}
    (junction 66) -> (junction 82) [order 2]
    (junction 66) -> (junction 69) [order 1] : [VVMC_MemoryShiftCount_enum < VVMC_RollAveCount_enum]
    (junction 82) -> (junction 80) : {VVMC_RollAveCount_enum = KVMC_RollAveLevel_enum}
    (junction 73) -> (junction 66) : {VVMC_MemoryShiftCount_enum++}
    (junction 69) -> (junction 71) : {VVMC_Memory_raw32[VVMC_MemoryShiftCount_enum] =...
        |  VVMC_Memory_raw32[VVMC_RollAveCount_enum - KVMC_RollAveLevel_enum + VVMC_MemoryShiftCount_enum]}
    (junction 25) -> (junction 14)
    (junction 71) -> (junction 73)
    (junction 80) -> (junction 78)
    (junction 45) -> (junction 39) [order 2]
    (junction 45) -> (junction 15) [order 1] : [VVMC_ShiftCount_enum < VVMC_RollAveCount_enum]
    (junction 41) -> (junction 45) : { VVMC_ShiftCount_enum++}
    (junction 15) -> (junction 38) : {% Gy Memory Shift
        |  VVMC_Memory_raw32[VVMC_ShiftCount_enum] = VVMC_Memory_raw32[VVMC_ShiftCount_enum + ONE_INT]}
    (junction 38) -> (junction 41)
  data: KVMC_RollAveLevel_enum input uint8; VVMC_ShiftCount_enum local uint8; VVMC_RollAveCount_enum local uint8; VVMC_Memory_raw32 local single size=256; ZERO_FLOAT input single; ONE_INT input uint8; VVMC_RollAve_raw32 output single; VINP_INPData_raw32 input single; VVMC_MemoryShiftCount_enum local uint8

== stateflow chart vmc/VMC/MSA function/MSAActivationHandshake/Chart ==
  state MSAActivationHandshake
    en:
    VVMC_MSACtrlSta_enum = ENUM_ADASMSASTA_OFF;
    VVMC_MSASpdWar_flg = FALSE;
    VVMC_MSAActive_flg = FALSE;
    VVMC_CheckMeterSpdLoop_flg = FALSE;
    VVMC_WaitResetSpdLoop_flg = FALSE; % detect set spd not in threshold
    state MSA_OFF
    state MSA_ERROR
    state MSA_DetectSpeed
      en:
      VVMC_CheckMeterSpdLoop_flg = FALSE;
      (default) -> (junction 89)
      (junction 89) -> (junction 90) [order 1] : [VVMC_MSASetSpd_kph >= VVMC_MSAActiveMetSpdLo_kph &&...
          |  VVMC_MSASetSpd_kph <=  KVMC_MSAActiveMetSpdHi_kph]
      (junction 89) -> (junction 91) [order 2]
      (junction 90) -> (junction 197)
      (junction 91) -> (junction 92) [order 1] : [VVMC_MSASetSpd_kph > KVMC_MSAActiveMetSpdHi_kph]
          | {VVMC_MSACtrlSta_enum = ENUM_ADASMSASTA_OVERSPEED;}
      (junction 91) -> (junction 93) [order 2]
      (junction 92) -> (junction 94)
      (junction 93) -> (junction 94) : %[VINP_SetSpd_kph < KVMC_MSAActiveMetSpdLo_kph]
          | {VVMC_MSACtrlSta_enum = ENUM_ADASMSASTA_UNDERSPEED;}
      (junction 94) -> (junction 96) : {VVMC_WaitResetSpdLoop_flg = TRUE;}
      MSA_DetectSpeed -> (junction 197) : [VVMC_CheckMeterSpdLoop_flg]{VVMC_CheckMeterSpdLoop_flg = FALSE;}
      (junction 197) -> (junction 191) [order 1] : [VINP_VehSpeed_kph >=VVMC_MSASpdBand_kph]
      (junction 191) -> (junction 221) : {VVMC_MSACtrlSta_enum = ENUM_ADASMSASTA_ACTIVE;
          | VVMC_MSAActive_flg = TRUE;}
      (junction 197) -> (junction 185) [order 2] : {VVMC_MSACtrlSta_enum = ENUM_ADASMSASTA_STANDBY;
          | VVMC_MSAActive_flg = FALSE;}
      (junction 221) -> (junction 217) [order 1] : [VVMC_MSAUnLimit_flg ||...
          | VVMC_AntiSpdLimEn_flg]
          | %add20231124
      (junction 217) -> (junction 257) [order 1] : [VVMC_AntiSpdLimEn_flg]
          | %add20240111
      (junction 221) -> (junction 219) [order 2]
      (junction 217) -> (junction 218) [order 2] : {VVMC_MSACtrlSta_enum = ENUM_ADASMSASTA_UNLIMIT;}
      (junction 257) -> (junction 258) : {VVMC_MSACtrlSta_enum = ENUM_ADASMSASTA_OFF;}
          | %add20240722
      (junction 218) -> (junction 219) : %add20231124
      (junction 258) -> (junction 218) : %add20230111
      (junction 219) -> (junction 189)
      (junction 189) -> (junction 186) [order 1] : [(VVMC_CalMeterSpeed_kph - VVMC_MSASetSpd_kph)...
          | >= KVMC_CCMSASpdWar_kph]
      (junction 189) -> (junction 196) [order 2] : {VVMC_MSASpdWar_flg = FALSE;}
      (junction 186) -> (junction 203) : {VVMC_MSASpdWar_flg = TRUE;}
      (junction 185) -> (junction 196)
      (junction 196) -> (junction 203)
      (junction 203) -> (junction 190) [order 1] : [((VVMC_MSASpdCtrlMode_enum != 3 && VVMC_MSASpdCtrlMode_enum != 4) ||...
          |   VVMC_DetectSWCCANCEL_flg) && !VVMC_AntiSpdLimEn_flg]
          | %add20231228
      (junction 203) -> (junction 230) [order 2]
      (junction 190) -> (junction 188) : {VVMC_MSAActive_flg = FALSE;
          | VVMC_MSACtrlSta_enum = ENUM_ADASMSASTA_OFF;
          | VVMC_MSASpdWar_flg = FALSE;
          | VVMC_MSASetCANCEL_flg = TRUE;}
          | %Back to outer first loop.
      (junction 230) -> (junction 232) [order 1] : [VINP_SWCResUpSta_flg || VINP_SWCSetdownSta_flg || VVMC_AntiSpdLimEn_flg]
          | %add20231229
      (junction 230) -> (junction 238) [order 2]
      (junction 232) -> (junction 233) : {VVMC_CheckMeterSpdLoop_flg = TRUE;
          | VVMC_MSASetCANCEL_flg = FALSE;}
          | %add20231201
      (junction 238) -> (junction 240) [order 1] : [VVMC_MSASetCANCEL_flg]
          | %add20231201
      (junction 238) -> (junction 199) [order 2] : {VVMC_CheckMeterSpdLoop_flg = TRUE;}
          | %add20231201
      (junction 240) -> (junction 242) : {VVMC_MSAActive_flg = FALSE;
          | VVMC_MSACtrlSta_enum = ENUM_ADASMSASTA_OFF;
          | VVMC_MSASpdWar_flg = FALSE;}
          | %Back to outer first loop
          | %add20231201
    state MSA_OFF1
    (default) -> (junction 73)
    MSAActivationHandshake -> (junction 73) [order 2] : [VVMC_MSACtrlSta_enum == ENUM_ADASMSASTA_OFF...
        |  || VVMC_MSACtrlSta_enum == ENUM_ADASMSASTA_ERROR]
    (junction 73) -> (junction 74) [order 1] : [VVMC_MSASpdCtrlMode_enum == 3 ||...
        | VVMC_MSASpdCtrlMode_enum == 4]
    (junction 74) -> (junction 75) [order 1] : [VTQD_ExternalTqAllow_flg]
    (junction 73) -> MSA_OFF [order 2] : {VVMC_MSACtrlSta_enum = ENUM_ADASMSASTA_OFF;
        |  VVMC_MSAActive_flg = FALSE;}
    (junction 74) -> MSA_ERROR [order 2] : {VVMC_MSACtrlSta_enum = ENUM_ADASMSASTA_ERROR;
        |  VVMC_MSAActive_flg = FALSE;}
    (junction 75) -> (junction 146)
    MSAActivationHandshake -> (junction 146) [order 1] : [VVMC_WaitResetSpdLoop_flg && VTQD_ExternalTqAllow_flg]{VVMC_WaitResetSpdLoop_flg = FALSE;}
    (junction 146) -> MSA_DetectSpeed [order 1] : [VVMC_MSASetSpd_kph!=ZERO_INT]
    (junction 146) -> MSA_OFF1 [order 2] : {VVMC_MSACtrlSta_enum = ENUM_ADASMSASTA_OFF;}
  (default) -> MSAActivationHandshake
  MSAActivationHandshake -> MSAActivationHandshake [order 1] : [!VTQD_ExternalTqAllow_flg || VTQD_GearActualPosn_enum != ENUM_GEARACTUALPOSN_D]
  data: VVMC_MSACtrlSta_enum output uint8; VVMC_MSASpdWar_flg output boolean; VVMC_MSAActive_flg output boolean; VVMC_MSASpdCtrlMode_enum input; VTQD_ExternalTqAllow_flg input; KVMC_MSAActiveMetSpdHi_kph input; VINP_VehSpeed_kph input; VVMC_MSAActiveMetSpdLo_kph input; VVMC_MSASetSpd_kph input; KVMC_CCMSASpdWar_kph input; VVMC_DetectSWCCANCEL_flg input; VVMC_MSASpdBand_kph input; VVMC_CheckMeterSpdLoop_flg local boolean; VVMC_WaitResetSpdLoop_flg local boolean; VVMC_MSAUnLimit_flg input; VTQD_GearActualPosn_enum input; ENUM_GEARACTUALPOSN_D parameter; VINP_SWCResUpSta_flg input; VINP_SWCSetdownSta_flg input; VVMC_MSASetCANCEL_flg local boolean; ENUM_ADASMSASTA_ERROR parameter; ENUM_ADASMSASTA_OFF parameter; FALSE parameter; ENUM_ADASMSASTA_ACTIVE parameter; ENUM_ADASMSASTA_OVERSPEED parameter; ENUM_ADASMSASTA_STANDBY parameter; ENUM_ADASMSASTA_UNDERSPEED parameter; ENUM_ADASMSASTA_UNLIMIT parameter; TRUE parameter; ZERO_INT parameter; VVMC_AntiSpdLimEn_flg input; VVMC_CalMeterSpeed_kph input

== stateflow chart vmc/VMC/Vehicle Speed Estimation/Scheduler ==
  state trigger_100ms
    (default) -> (junction 1) : {
        | counter = 0;
        | }
    trigger_100ms -> (junction 1) : {
        | counter++;
        | }
    (junction 1) -> (junction 8) [order 1] : [counter%%uint8((10/task_time_s)) == 0]  /* 10s trigger */
    (junction 1) -> (junction 5) [order 2]
    (junction 8) -> (junction 9) : {
        | trig_KF_10s;
        | counter = 0;
        | }
    (junction 9) -> (junction 5)
  data: counter local uint32 size=1; task_time_s input
  events: trig_KF_10s output FUNCTION_CALL_EVENT

== stateflow chart vmc/VMC/CruiseControlFunction/CCActiveDetermination/Chart ==
  state CCActiveDetermination
    (default) -> (junction 141) : {
        |  VVMC_CCCtrlSta_enum = 0;
        |  VVMC_CruzActive_flg = FALSE;
        |  VVMC_CCSpdWar_flg = FALSE;
        |  VVMC_SWCSetDownLoop_flg = FALSE;
        |  VVMC_CruzLoopSpdChk_flg = FALSE;
        |  VVMC_CruzReActiveLoop_flg = FALSE;
        |  VVMC_CruzLoopNOSpdChk_flg = FALSE;
        |  VVMC_WaitingCmdLoop_flg = FALSE;
        |  }
    CCActiveDetermination -> (junction 141) [order 5]
    (junction 141) -> (junction 123) [order 1] : [VINP_ZoneSpdCrlMode_enum == 2]
    (junction 141) -> (junction 152) [order 2] : {VVMC_CCCtrlSta_enum = 0;
        | VVMC_CruzActive_flg = FALSE;}
        | %Back to first loop
        | %add20230706
    (junction 123) -> (junction 122)
    (junction 122) -> (junction 136) [order 1] : [VTQD_ExternalTqAllow_flg]
    (junction 122) -> (junction 294) [order 2] : {VVMC_CCCtrlSta_enum = 5;
        | VVMC_CruzActive_flg = FALSE;}
        | %Back to first loop
        | %add20230706
    (junction 136) -> (junction 229)
    CCActiveDetermination -> (junction 229) [order 4] : [VVMC_SWCSetDownLoop_flg && VTQD_ExternalTqAllow_flg]{VVMC_SWCSetDownLoop_flg = FALSE;} %add0230705
    (junction 229) -> (junction 145) : {VVMC_CCCtrlSta_enum = 1;}
    (junction 145) -> (junction 154) [order 1] : [VVMC_DetectSWCSetDown_flg || VVMC_DetectSWCResUp_flg]
    (junction 145) -> (junction 158) [order 2] : %Back to first loop
    (junction 154) -> (junction 156)
    CCActiveDetermination -> (junction 156) [order 3] : [(VVMC_CruzLoopSpdChk_flg || VVMC_CruzReActiveLoop_flg)...
        | && VTQD_ExternalTqAllow_flg]
        | {VVMC_CruzLoopSpdChk_flg = FALSE;
        | VVMC_CruzReActiveLoop_flg = FALSE;} %add20230711
    (junction 156) -> (junction 160) [order 1] : [VINP_SetSpd_kph >= KVMC_CCActiveMetSpdLo_kph &&...
        |  VINP_SetSpd_kph <=  KVMC_CCActiveMetSpdHi_kph &&...
        |  VINP_VehSpeed_kph >= KVMC_CCModeEnSpd_kph]
    (junction 156) -> (junction 162) [order 2]
    (junction 160) -> (junction 234)
    (junction 162) -> (junction 164) [order 1] : [VINP_SetSpd_kph < KVMC_CCActiveMetSpdLo_kph]
    (junction 162) -> (junction 166) [order 2] : {VVMC_CCCtrlSta_enum = 1;}
        | %TBD
        | %add20230711
    (junction 164) -> (junction 168) : {VVMC_CCCtrlSta_enum = 1;}
        | %TBD
        | %add20230711
    (junction 168) -> (junction 166)
    (junction 166) -> (junction 232) : {VVMC_SWCSetDownLoop_flg = TRUE;}
    (junction 234) -> (junction 238) : {VVMC_CruzActive_flg = TRUE;
        |  VVMC_CCCtrlSta_enum = 2;}
    CCActiveDetermination -> (junction 238) [order 2] : [VVMC_CruzLoopNOSpdChk_flg && VTQD_ExternalTqAllow_flg]{VVMC_CruzLoopNOSpdChk_flg = FALSE;} %add20230705
    (junction 238) -> (junction 236) [order 1] : [(VVMC_CalMeterSpeed_kph - VINP_SetSpd_kph) >=...
        |  KVMC_CCMSASpdWar_kph]
    (junction 238) -> (junction 240) [order 2] : {VVMC_CCSpdWar_flg = FALSE;}
    (junction 236) -> (junction 242) : {VVMC_CCSpdWar_flg = TRUE;}
    (junction 242) -> (junction 240)
    (junction 240) -> (junction 305)
    (junction 305) -> (junction 311) [order 1] : [VVMC_CCPedalOvrd_flg]
    (junction 305) -> (junction 307) [order 2] : {VVMC_CCCtrlSta_enum = 2}
    (junction 311) -> (junction 313) : {VVMC_CCCtrlSta_enum = 7}
    (junction 313) -> (junction 307)
    (junction 307) -> (junction 245)
    (junction 245) -> (junction 247) [order 1] : [ VINP_ZoneSpdCrlMode_enum != 2 ||...
        |   VVMC_DetectSWCCANCEL_flg ||...
        |   VINP_BrkSwSta_flg ||...
        |   VINP_BrakeSWGPIO_flg ||...
        |   VINP_BrkPedalPos_pct >= KVMC_CCDisBrkPos_pct]
    (junction 245) -> (junction 249) [order 2] : {VVMC_CruzLoopNOSpdChk_flg = TRUE;}
    (junction 247) -> (junction 297) : {VVMC_CCSpdWar_flg = FALSE;}
    CCActiveDetermination -> (junction 297) [order 1] : [VVMC_WaitingCmdLoop_flg && VTQD_ExternalTqAllow_flg]{VVMC_WaitingCmdLoop_flg = FALSE;} %add20230705
    (junction 297) -> (junction 254) [order 1] : [ VINP_ZoneSpdCrlMode_enum == 2 ]
    (junction 297) -> (junction 258) [order 2] : {VVMC_CruzActive_flg = FALSE;
        |  VVMC_CCCtrlSta_enum = 0;}
        | %Back to first loop
    (junction 254) -> (junction 256) : {VVMC_CruzActive_flg = FALSE;
        |  VVMC_CCCtrlSta_enum = 1;}
    (junction 256) -> (junction 261) [order 1] : [VVMC_DetectSWCResUp_flg]
    (junction 256) -> (junction 263) [order 2]
    (junction 261) -> (junction 265) : {VVMC_CruzReActiveLoop_flg = TRUE;}
    (junction 263) -> (junction 267) [order 1] : [VVMC_DetectSWCSetDown_flg]
    (junction 263) -> (junction 269) [order 2] : {VVMC_WaitingCmdLoop_flg = TRUE;}
    (junction 267) -> (junction 271) : {VVMC_CruzLoopSpdChk_flg = TRUE;}
  CCActiveDetermination -> CCActiveDetermination [order 1] : [!VTQD_ExternalTqAllow_flg  || VTQD_GearActualPosn_enum != ENUM_GEARACTUALPOSN_D || !VTQD_ExtDoorAllow_flg]
  data: VVMC_CCCtrlSta_enum output uint8; VVMC_CCSpdWar_flg output boolean; VVMC_CruzActive_flg output boolean; VINP_ZoneSpdCrlMode_enum input; VTQD_ExternalTqAllow_flg input; VVMC_DetectSWCSetDown_flg input; KVMC_CCActiveMetSpdHi_kph input; VINP_VehSpeed_kph input; KVMC_CCActiveMetSpdLo_kph input; VINP_SetSpd_kph input; KVMC_CCMSASpdWar_kph input; VINP_BrakeSWGPIO_flg input; VVMC_DetectSWCCANCEL_flg input; VINP_BrkSwSta_flg input; VVMC_DetectSWCResUp_flg input; VVMC_CruzLoopNOSpdChk_flg local boolean; VVMC_CruzLoopSpdChk_flg local boolean; VVMC_WaitingCmdLoop_flg local boolean; VVMC_SWCSetDownLoop_flg local boolean; VVMC_CruzReActiveLoop_flg local boolean; VVMC_CCPedalOvrd_flg input; VTQD_GearActualPosn_enum input; VINP_BrkPedalPos_pct input; ENUM_GEARACTUALPOSN_D parameter; KVMC_CCDisBrkPos_pct input; KVMC_CCModeEnSpd_kph input; FALSE parameter; TRUE parameter; VTQD_ExtDoorAllow_flg input; VVMC_CalMeterSpeed_kph input

== stateflow chart vmc/VMC/IMU/IMU sensing result /RollingAverage ==
  state RollingAverage
    (default) -> (junction 2) : {VVMC_RollAveCount_enum = ONE_INT}
    RollingAverage -> (junction 2)
    (junction 2) -> (junction 3) : {VVMC_RollAve_raw32 = ZERO_FLOAT}
    (junction 3) -> (junction 100) [order 1] : [VVMC_RollAveCount_enum < KVMC_RollAveLevel_enum]
    (junction 3) -> (junction 37) [order 2]
    (junction 100) -> (junction 5) : {% Memory
        |  VVMC_Memory_raw32[VVMC_RollAveCount_enum] = VINP_INPData_raw32;
        |
        |  % Memory Shift Counter
        |  VVMC_ShiftCount_enum = ONE_INT}
    (junction 5) -> (junction 7) [order 2]
    (junction 5) -> (junction 6) [order 1] : [VVMC_ShiftCount_enum <= VVMC_RollAveCount_enum]
    (junction 7) -> (junction 8) : {% Rolling Average
        |  VVMC_RollAve_raw32 = VVMC_RollAve_raw32 / VVMC_RollAveCount_enum;
        |
        |  % Rolling Average Counter
        |  VVMC_RollAveCount_enum++}
    (junction 35) -> (junction 5) : {VVMC_ShiftCount_enum++}
    (junction 6) -> (junction 36) : {% Rolling Average Sum
        |  VVMC_RollAve_raw32 = VVMC_RollAve_raw32 + VVMC_Memory_raw32[VVMC_ShiftCount_enum];
        |  }
    (junction 36) -> (junction 35)
    (junction 37) -> (junction 76) [order 1] : [VVMC_RollAveCount_enum == KVMC_RollAveLevel_enum]
    (junction 76) -> (junction 47)
    (junction 37) -> (junction 60) [order 2]
    (junction 78) -> (junction 76)
    (junction 47) -> (junction 30) : {% Memory
        |  VVMC_Memory_raw32[VVMC_RollAveCount_enum] = VINP_INPData_raw32;
        |
        |  % Memory Shift Counter
        |  VVMC_ShiftCount_enum = ONE_INT;
        | }
    (junction 60) -> (junction 62) [order 1] : [VVMC_RollAveCount_enum > KVMC_RollAveLevel_enum]
    (junction 60) -> (junction 39) [order 2]
    (junction 62) -> (junction 66) : {VVMC_MemoryShiftCount_enum = ONE_INT}
    (junction 30) -> (junction 48) [order 2]
    (junction 30) -> (junction 22) [order 1] : [VVMC_ShiftCount_enum <= VVMC_RollAveCount_enum]
    (junction 48) -> (junction 45) : {% Rolling Average
        |  VVMC_RollAve_raw32 = VVMC_RollAve_raw32 / VVMC_RollAveCount_enum;
        |
        |  % Memory Shift Counter
        |  VVMC_ShiftCount_enum = ONE_INT}
    (junction 14) -> (junction 30) : {VVMC_ShiftCount_enum++}
    (junction 22) -> (junction 25) : {% Rolling Average Sum
        |  VVMC_RollAve_raw32 = VVMC_RollAve_raw32 + VVMC_Memory_raw32[VVMC_ShiftCount_enum]}
    (junction 66) -> (junction 82) [order 2]
    (junction 66) -> (junction 69) [order 1] : [VVMC_MemoryShiftCount_enum < VVMC_RollAveCount_enum]
    (junction 82) -> (junction 80) : {VVMC_RollAveCount_enum = KVMC_RollAveLevel_enum}
    (junction 73) -> (junction 66) : {VVMC_MemoryShiftCount_enum++}
    (junction 69) -> (junction 71) : {VVMC_Memory_raw32[VVMC_MemoryShiftCount_enum] =...
        |  VVMC_Memory_raw32[VVMC_RollAveCount_enum - KVMC_RollAveLevel_enum + VVMC_MemoryShiftCount_enum]}
    (junction 25) -> (junction 14)
    (junction 71) -> (junction 73)
    (junction 80) -> (junction 78)
    (junction 45) -> (junction 39) [order 2]
    (junction 45) -> (junction 15) [order 1] : [VVMC_ShiftCount_enum < VVMC_RollAveCount_enum]
    (junction 41) -> (junction 45) : { VVMC_ShiftCount_enum++}
    (junction 15) -> (junction 38) : {% Gy Memory Shift
        |  VVMC_Memory_raw32[VVMC_ShiftCount_enum] = VVMC_Memory_raw32[VVMC_ShiftCount_enum + ONE_INT]}
    (junction 38) -> (junction 41)
  data: KVMC_RollAveLevel_enum input uint8; VVMC_ShiftCount_enum local uint8; VVMC_RollAveCount_enum local uint8 [..100]; VVMC_Memory_raw32 local single size=256; ZERO_FLOAT input single; ONE_INT input uint8; VVMC_RollAve_raw32 output single; VINP_INPData_raw32 input single; VVMC_MemoryShiftCount_enum local uint8

== stateflow chart vmc/VMC/Scheduler ==
  state Scheduler
    (default) -> (junction 3) : {counter = 0;}
    Scheduler -> (junction 3) : {counter++}
    (junction 3) -> (junction 5) [order 1] : [counter%%2 == 0]
    (junction 3) -> (junction 11) [order 2]
    (junction 5) -> (junction 7) : {Trigger_10ms_1;
        |  counter = 0;}
    (junction 7) -> (junction 11)
  data: counter local uint8
  events: Trigger_10ms_1 output FUNCTION_CALL_EVENT
